simulink model "sigmadelta"  (Simulink 7.4)
settings: Solver=ode45  StartTime=0.0  StopTime=1000.0  RelTol=1e-3
libraries: simulink x2, dspsrcs4 x1, dspmlti4 x1
settings Model: Creator=Tibor  LastModifiedBy=Tibor

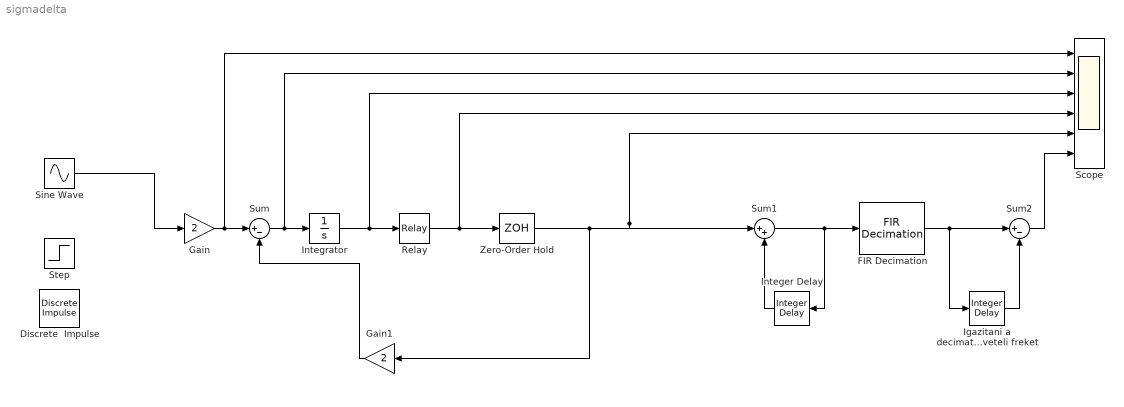
== system sigmadelta ==
  Discrete  Impulse : dspsrcs4/Discrete  Impulse  Delay=0  SampleTime=1  FrameSample=1  dataType=double  isSigned=on  wordLen=16  udDataType=sfix(16)  fracBitsMode=Best precision  numFracBits=15
  FIR Decimation : dspmlti4/FIR Decimation  DialogController=dspdialog.FIRDecimation  DialogControllerArgs=DataTag0  h=fir1(35,0.4)  D=5  filtStruct=Direct form  framing=Maintain input frame size  outputBufInitCond=0  roundingMode=Floor  overflowMode=off  FilterSource=Specify via dialog  FilterObject=Hm_firdecim
  Gain : Gain  Gain=2  ParameterDataType=fixdt(1, 16)  ParameterScaling=2^0  OutDataType=fixdt(1, 16)  OutScaling=2^0
  Gain1 : Gain  Gain=2  ParameterDataType=fixdt(1, 16)  ParameterScaling=2^0  OutDataType=fixdt(1, 16)  OutScaling=2^0
  Igazitani a decimatorhoz a mintaveteli freket : simulink/Discrete/Integer Delay  vinit=0.0  samptime=5  NumDelays=5
  Integer Delay : simulink/Discrete/Integer Delay  vinit=0.0  samptime=-1  NumDelays=1
  Integrator : Integrator
  Relay : Relay  OnSwitchValue=0  OffSwitchValue=0  OffOutputValue=-1  OutDataType=fixdt(1, 16)  OutScaling=2^0
  Scope : Scope  NumInputPorts=6
      settings: YMin=-5~-5~-5~-5~-5~-50  YMax=5~5~5~5~5~50  SampleInput=on
  Sine Wave : Sin  Amplitude=1  Bias=0  Frequency=0.01  Phase=0  Samples=10  SampleTime=0  Offset=0
  Step : Step  SampleTime=0
  Sum : Sum  Inputs=|+-  OutDataType=fixdt(1, 16)  OutScaling=2^0
  Sum1 : Sum  Inputs=|++  OutDataType=fixdt(1, 16)  OutScaling=2^0
  Sum2 : Sum  Inputs=|+-  OutDataType=fixdt(1, 16)  OutScaling=2^0
  Zero-Order Hold : ZeroOrderHold
  wires:
  Gain/1 -> Sum/1, Scope/1
  Sum/1 -> Integrator/1, Scope/2
  Integrator/1 -> Relay/1, Scope/3
  Zero-Order Hold/1 -> Gain1/1, Scope/5, Sum1/1
  Gain1/1 -> Sum/2
  Relay/1 -> Zero-Order Hold/1, Scope/4
  Integer Delay/1 -> Sum1/2
  Sum1/1 -> Integer Delay/1, FIR Decimation/1
  Igazitani a decimatorhoz a mintaveteli freket/1 -> Sum2/2
  FIR Decimation/1 -> Sum2/1, Igazitani a decimatorhoz a mintaveteli freket/1
  Sum2/1 -> Scope/6
  Sine Wave/1 -> Gain/1
